simulink model "dc_motor_sim"  (R2021a)
settings: Solver=VariableStepAuto  StartTime=0.0  StopTime=8  FixedStep=1e-3  MaxStep=10e-5  RelTol=1e-3
libraries: spsThyristorLib x4, spsVoltageMeasurementLib x3, spspowerguiLib x2, simulink x2, spsSeriesRLCBranchLib x1, spsACVoltageSourceLib x1, dspswit3 x1, spsUniversalBridgeLib x1
settings Model: Creator=AHMED  LastModifiedBy=AHMED

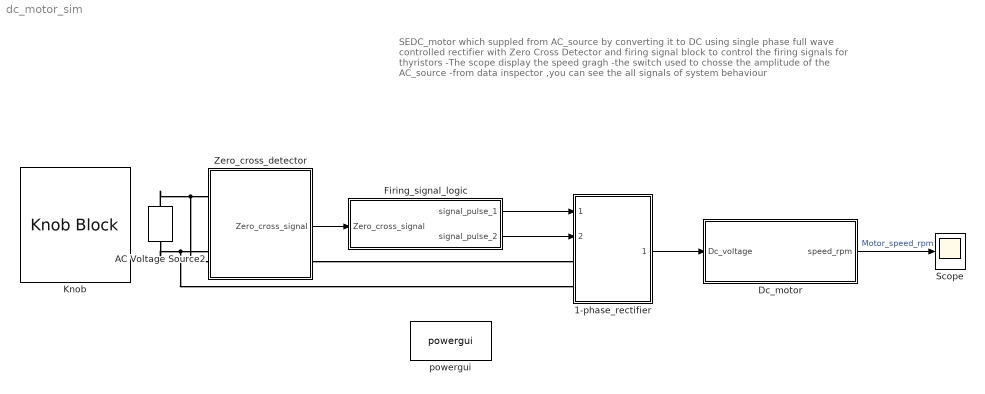
== system dc_motor_sim ==
  note: SEDC_motor which suppled from AC_source by converting it to DC using single phase full wave controlled rectifier with Zero Cross Detector and firing signal block to control the firing signals for thyristors
      | -The scope display the speed gragh
      | -the switch used to chosse the amplitude of the AC_source
      | -from data inspector ,you can see the all signals of system behaviour
  1-phase_rectifier : Subsystem
  AC Voltage Source2 : spsACVoltageSourceLib/AC Voltage Source  Amplitude=220  Phase=0  Frequency=50  SampleTime=0  Measurements=None  BusType=swing  Pref=10e3  Qref=0  Qmin=-inf  Qmax=+inf
  Dc_motor : Subsystem  mask{Ra=0.5, La=0.1, Km=1.6, Kb=1.6, Tl=100, J=5, B=0.01}
  Firing_signal_logic : Subsystem  mask{firing_angle=30}
      mask prompts: firing_angle "firing_angle(deg)"
  Knob : KnobBlock  ScaleMax=380
  Scope : Scope
  Zero_cross_detector : Subsystem
  powergui : spspowerguiLib/powergui  Priority=1  SimulationMode=Continuous  SampleTime=50e-6  frequency=60  Iterations=50  frequencyindice=0  Pbase=100e6  ErrMax=1e-4  UnitsV=kV  UnitsW=MW  buscounter=0  FunctionMessages=off  echomessages=off  EnableUseOfTLC=off  CurrentSourceSwitches=off  DisableSnubberDevices=off  DisableRonSwitches=off  DisableVfSwitches=off  DisplayEquations=off  AutomaticDiscreteSolvers=off  SolverType=Tustin/Backward Euler (TBE)  Interpol=off  ExternalGateDelay=off  methode=off  Ts=100  x0status=blocks  SPID=on  SwTol=0  HookPort=off  NonlinearTolerance=1e-4  nMaxIteration=100  ContinueOnMaxIteration=off  RestoreLinks=warning  ResistiveCurrentMeasurement=off  Frange=[0:2:500]  Ylog=off  Xlog=on  ShowGrid=off  save=off  variable=ZData  structure=0  ZoomFFT=off  StartTime=0.0  cycles=1  DisplayStyle=1  fundamental=60  FreqAxis=off  MaxFrequency=1000  frequencyindicesteady=1  RmsSteady=1  display=off
  wires:
  Dc_motor/1(speed_rpm) -> Scope/1  "Motor_speed_rpm"
  Zero_cross_detector/1(Zero_cross_signal) -> Firing_signal_logic/1(Zero_cross_signal)
  Firing_signal_logic/1(signal_pulse_1) -> 1-phase_rectifier/1(signal_pulse_1)
  Firing_signal_logic/2(signal_pulse_2) -> 1-phase_rectifier/2(signal_pulse_2)
  1-phase_rectifier/1(dc_voltage) -> Dc_motor/1(Dc_voltage)
  connections:
  AC Voltage Source2/RConn1 -- 1-phase_rectifier/LConn1 -- Zero_cross_detector/LConn1
  AC Voltage Source2/LConn1 -- 1-phase_rectifier/LConn2 -- Zero_cross_detector/LConn2

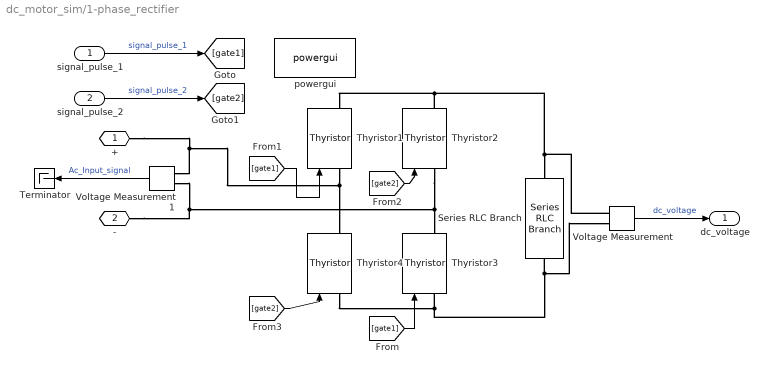
== system dc_motor_sim/1-phase_rectifier ==
  signal_pulse_1 : Inport
  signal_pulse_2 : Inport  Port=2
  Series RLC Branch : spsSeriesRLCBranchLib/Series RLC Branch  LConnTagsString=__new0  RConnTagsString=__new0  BranchType=R  Resistance=50  Inductance=1e-3  SetiL0=off  InitialCurrent=0  Capacitance=1e-6  Setx0=off  InitialVoltage=0  Measurements=Branch voltage
  Terminator : Terminator
  Thyristor{1..4} (4 alike) : spsThyristorLib/Thyristor  Ron=0.001  Lon=0  Vf=0.8  IC=0  Rs=500  Cs=250e-9  Measurements=on
  Voltage Measurement : spsVoltageMeasurementLib/Voltage Measurement  PhasorSimulation=off  OutputType=Complex  PSBequivalent=0
  Voltage Measurement1 : spsVoltageMeasurementLib/Voltage Measurement  PhasorSimulation=off  OutputType=Complex  PSBequivalent=0
  powergui : spspowerguiLib/powergui  Priority=1  SimulationMode=Continuous  SampleTime=50e-6  frequency=60  Iterations=50  frequencyindice=0  Pbase=100e6  ErrMax=1e-4  UnitsV=kV  UnitsW=MW  buscounter=0  FunctionMessages=off  echomessages=off  EnableUseOfTLC=off  CurrentSourceSwitches=off  DisableSnubberDevices=off  DisableRonSwitches=off  DisableVfSwitches=off  DisplayEquations=off  AutomaticDiscreteSolvers=off  SolverType=Tustin/Backward Euler (TBE)  Interpol=off  ExternalGateDelay=off  methode=off  Ts=100  x0status=blocks  SPID=on  SwTol=0  HookPort=off  NonlinearTolerance=1e-4  nMaxIteration=100  ContinueOnMaxIteration=off  RestoreLinks=warning  ResistiveCurrentMeasurement=off  Frange=[0:2:500]  Ylog=off  Xlog=on  ShowGrid=off  save=off  variable=ZData  structure=0  ZoomFFT=off  StartTime=0.0  cycles=1  DisplayStyle=1  fundamental=60  FreqAxis=off  MaxFrequency=1000  frequencyindicesteady=1  RmsSteady=1  display=off
  + : PMIOPort  Side=Left
  - : PMIOPort  Port=2  Side=Left
  dc_voltage : Outport
  wires:
  signal_pulse_1/1 -> [gate1]  "signal_pulse_1"
  signal_pulse_2/1 -> [gate2]  "signal_pulse_2"
  [gate1] -> Thyristor1/1
  [gate2] -> Thyristor4/1
  [gate1] -> Thyristor3/1
  [gate2] -> Thyristor2/1
  Voltage Measurement1/1 -> Terminator/1  "Ac_Input_signal"
  Voltage Measurement/1 -> dc_voltage/1  "dc_voltage"
  connections:
  Thyristor4/LConn1 -- Series RLC Branch/RConn1 -- Voltage Measurement/LConn2 -- Thyristor3/LConn1
  Voltage Measurement/LConn1 -- Series RLC Branch/LConn1 -- Thyristor2/RConn1 -- Thyristor1/RConn1
  Thyristor2/LConn1 -- -/RConn1 -- Voltage Measurement1/LConn2 -- Thyristor3/RConn1
  Thyristor1/LConn1 -- +/RConn1 -- Voltage Measurement1/LConn1 -- Thyristor4/RConn1

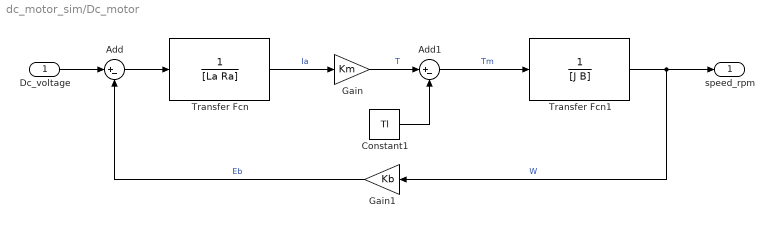
== system dc_motor_sim/Dc_motor ==
  Dc_voltage : Inport
  Add : Sum  Inputs=|+-
  Add1 : Sum  Inputs=|+-
  Constant1 : Constant  Value=Tl
  Gain : Gain  Gain=Km
  Gain1 : Gain  Gain=Kb
  Transfer Fcn : TransferFcn  Denominator=[La Ra]
  Transfer Fcn1 : TransferFcn  Denominator=[J B]
  speed_rpm : Outport
  wires:
  Constant1/1 -> Add1/2
  Add1/1 -> Transfer Fcn1/1  "Tm"
  Transfer Fcn/1 -> Gain/1  "Ia"
  Gain1/1 -> Add/2  "Eb"
  Gain/1 -> Add1/1  "T"
  Add/1 -> Transfer Fcn/1
  Transfer Fcn1/1 -> speed_rpm/1, Gain1/1  "W"
  Dc_voltage/1 -> Add/1

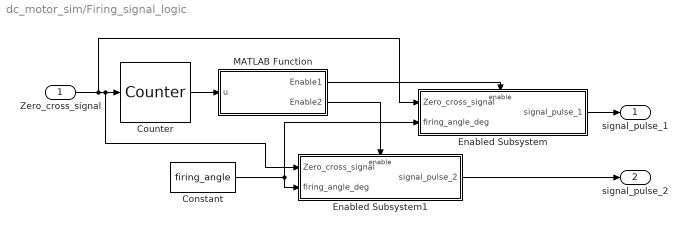
== system dc_motor_sim/Firing_signal_logic ==
  Zero_cross_signal : Inport
  Constant : Constant  Value=firing_angle
  Counter : dspswit3/Counter  Direction=Up  CountEvent=Rising edge  CounterSize=User defined  MaxCount=255  InitialCount=0  Output=Count  HitValue=32  ResetInput=off  SamplesPerFrame=1  Ts=1  CntDtype=double  HitDtype=Logical
  Enabled Subsystem : Subsystem  TreatAsAtomicUnit=on
  Enabled Subsystem1 : Subsystem  TreatAsAtomicUnit=on
  MATLAB Function : MATLAB Function  TreatAsAtomicUnit=on
  signal_pulse_1 : Outport
  signal_pulse_2 : Outport  Port=2
  wires:
  Zero_cross_signal/1 -> Enabled Subsystem1/1(Zero_cross_signal), Counter/1, Enabled Subsystem/1(Zero_cross_signal)
  Counter/1 -> MATLAB Function/1(u)
  MATLAB Function/1(Enable1) -> Enabled Subsystem/Enable
  MATLAB Function/2(Enable2) -> Enabled Subsystem1/Enable
  Constant/1 -> Enabled Subsystem/2(firing_angle_deg), Enabled Subsystem1/2(firing_angle_deg)
  Enabled Subsystem/1(signal_pulse_1) -> signal_pulse_1/1
  Enabled Subsystem1/1(signal_pulse_2) -> signal_pulse_2/1

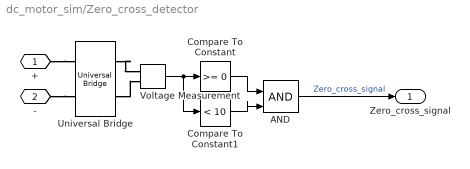
== system dc_motor_sim/Zero_cross_detector ==
  AND : Logic  IconShape=distinctive  AllPortsSameDT=off  OutDataTypeStr=boolean
  Compare To Constant : simulink/Logic and Bit Operations/Compare To Constant  relop=>=  const=0  OutDataTypeStr=boolean
  Compare To Constant1 : simulink/Logic and Bit Operations/Compare To Constant  relop=<  const=10  OutDataTypeStr=boolean
  Universal Bridge : spsUniversalBridgeLib/Universal Bridge  Arms=2  SnubberResistance=1e5  SnubberCapacitance=inf  Device=Diodes  Ron=1e-3  Lon=0  ForwardVoltages="[  0  0  ]"  ForwardVoltage=0  GTOparameters=[ 10e-6 , 20e-6 ]  IGBTparameters=[ 1e-6 , 2e-6 ]  Measurements=None  Measurements_2=None  converterType=Rectifier
  Voltage Measurement : spsVoltageMeasurementLib/Voltage Measurement  PhasorSimulation=off  OutputType=Complex  PSBequivalent=0
  + : PMIOPort  Side=Left
  - : PMIOPort  Port=2  Side=Left
  Zero_cross_signal : Outport
  wires:
  Voltage Measurement/1 -> Compare To Constant/1, Compare To Constant1/1
  Compare To Constant/1 -> AND/1
  Compare To Constant1/1 -> AND/2
  AND/1 -> Zero_cross_signal/1  "Zero_cross_signal"
  connections:
  +/RConn1 -- Universal Bridge/LConn1
  -/RConn1 -- Universal Bridge/LConn2
  Universal Bridge/RConn1 -- Voltage Measurement/LConn1
  Universal Bridge/RConn2 -- Voltage Measurement/LConn2

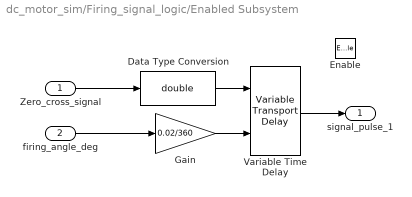
== system dc_motor_sim/Firing_signal_logic/Enabled Subsystem ==
  Zero_cross_signal : Inport
  firing_angle_deg : Inport  Port=2
  Enable : EnablePort
  Data Type Conversion : DataTypeConversion  OutDataTypeStr=double
  Gain : Gain  Gain=0.02/360
  Variable Time Delay : VariableTransportDelay  MaximumDelay=10
  signal_pulse_1 : Outport
  wires:
  Zero_cross_signal/1 -> Data Type Conversion/1
  firing_angle_deg/1 -> Gain/1
  Gain/1 -> Variable Time Delay/2
  Data Type Conversion/1 -> Variable Time Delay/1
  Variable Time Delay/1 -> signal_pulse_1/1

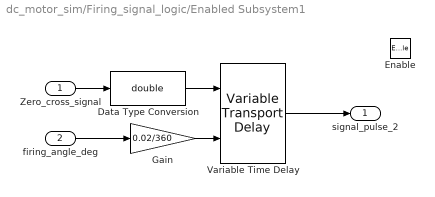
== system dc_motor_sim/Firing_signal_logic/Enabled Subsystem1 ==
  Zero_cross_signal : Inport
  firing_angle_deg : Inport  Port=2
  Enable : EnablePort
  Data Type Conversion : DataTypeConversion  OutDataTypeStr=double
  Gain : Gain  Gain=0.02/360
  Variable Time Delay : VariableTransportDelay  MaximumDelay=10
  signal_pulse_2 : Outport
  wires:
  Zero_cross_signal/1 -> Data Type Conversion/1
  Data Type Conversion/1 -> Variable Time Delay/1
  firing_angle_deg/1 -> Gain/1
  Gain/1 -> Variable Time Delay/2
  Variable Time Delay/1 -> signal_pulse_2/1

== matlab function dc_motor_sim/Firing_signal_logic/MATLAB Function ==
  data: u input; Enable1 output; Enable2 output
function [Enable1,Enable2] = fcn(u)
Enable1=0;
Enable2=0;

if mod(u,2)==0
    Enable1=1;
    Enable2=0;
end

if mod(u,2)==1
    Enable1=0;
    Enable2=1;
end
